simulink model "normal_feedback"  (R2016b)
settings: Solver=VariableStepAuto  StartTime=0.0  StopTime=10.0  RelTol=1e-3
undefined symbols (not defined in the file): A, B, C, k
settings Model: Creator=Amin  LastModifiedBy=Amin

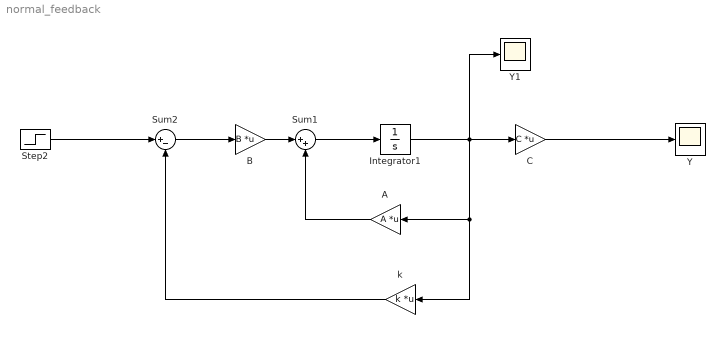
== system normal_feedback ==
  A : Gain  Gain=A  Multiplication=Matrix(K*u)
  B : Gain  Gain=B  Multiplication=Matrix(K*u)
  C : Gain  Gain=C  Multiplication=Matrix(K*u)
  Integrator1 : Integrator  InitialCondition=[0.3 0 0 0]
  Step2 : Step  After=0  SampleTime=0
  Sum1 : Sum  Inputs=|++
  Sum2 : Sum  Inputs=|+-
  Y : Scope
  Y1 : Scope
  k : Gain  Gain=k  Multiplication=Matrix(K*u)
  wires:
  C/1 -> Y/1
  Integrator1/1 -> Y1/1, C/1, k/1, A/1
  A/1 -> Sum1/2
  Sum1/1 -> Integrator1/1
  B/1 -> Sum1/1
  Step2/1 -> Sum2/1
  Sum2/1 -> B/1
  k/1 -> Sum2/2
